simulink model "lab1_SimulinkExtendedStateEstimator"  (R2020b)
settings: Solver=VariableStepAuto  StartTime=0.0  StopTime=10.0  RelTol=1e-3
undefined symbols (not defined in the file): A_hat_e, A_r, A_r_2, A_r_3, B_e, C_p, enable_Reference, K, L_e, sens, w_1, w_2
settings Model: Creator=Musta  LastModifiedBy=Musta

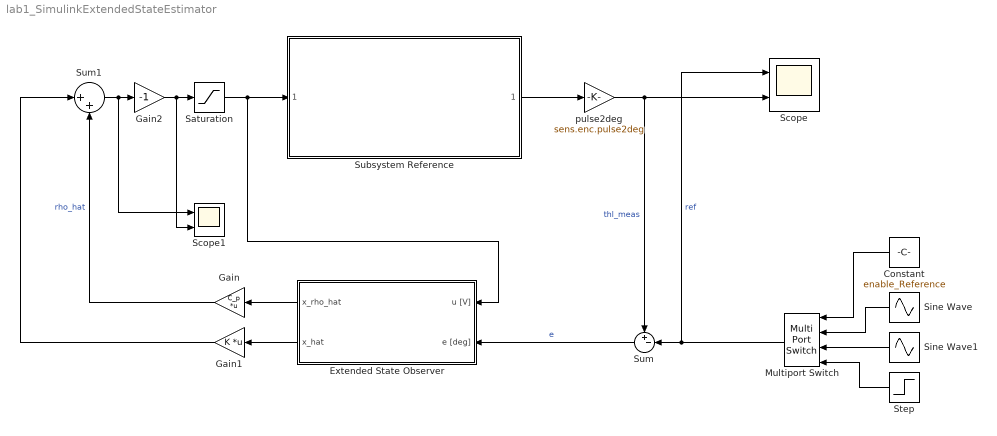
== system lab1_SimulinkExtendedStateEstimator ==
  Constant : Constant  Value=enable_Reference
  Extended State Observer : Subsystem
  Gain : Gain  Gain=C_p  Multiplication=Matrix(K*u)
  Gain1 : Gain  Gain=K  Multiplication=Matrix(K*u)
  Gain2 : Gain  Gain=-1
  Multiport Switch : MultiPortSwitch
  Saturation : Saturate  UpperLimit=10  LowerLimit=-10
  Scope : Scope  NumInputPorts=2
  Scope1 : Scope  NumInputPorts=2
  Sine Wave : Sin  Amplitude=A_r  Frequency=w_1  SampleTime=0
  Sine Wave1 : Sin  Amplitude=A_r_2  Frequency=w_2  SampleTime=0
  Step : Step  Time=0  After=A_r_3  SampleTime=0
  Subsystem Reference : Subsystem  ReferencedSubsystem=plant_Model
  Sum : Sum  Inputs=+-|
  Sum1 : Sum  Inputs=|++
  pulse2deg : Gain  Gain=sens.enc.pulse2deg
  wires:
  Multiport Switch/1 -> Scope/1, Sum/2  "ref"
  Sum1/1 -> Gain2/1, Scope1/1
  Sum/1 -> Extended State Observer/2(e [deg])  "e"
  pulse2deg/1 -> Sum/1, Scope/2  "thl_meas"
  Extended State Observer/1(x_rho_hat) -> Gain/1
  Gain/1 -> Sum1/2  "rho_hat"
  Extended State Observer/2(x_hat) -> Gain1/1
  Gain1/1 -> Sum1/1
  Saturation/1 -> Subsystem Reference/1, Extended State Observer/1(u [V])
  Gain2/1 -> Scope1/2, Saturation/1
  Subsystem Reference/1 -> pulse2deg/1
  Sine Wave/1 -> Multiport Switch/2
  Sine Wave1/1 -> Multiport Switch/3
  Step/1 -> Multiport Switch/4
  Constant/1 -> Multiport Switch/1

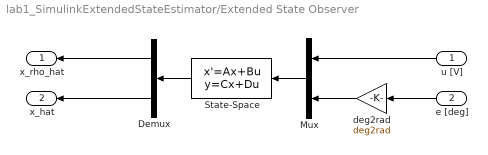
== system lab1_SimulinkExtendedStateEstimator/Extended State Observer ==
  u [V] : Inport
  e [deg] : Inport  Port=2
  Demux : Demux  Outputs=[3,2]
  Mux : Mux  Inputs=[1,1]
  State-Space : StateSpace  A=A_hat_e  B=[B_e L_e]  C=eye(5)  D=zeros(5,2)  InitialCondition=0
  deg2rad : Gain  Gain=deg2rad
  x_rho_hat : Outport
  x_hat : Outport  Port=2
  wires:
  e [deg]/1 -> deg2rad/1
  Demux/2 -> x_hat/1
  deg2rad/1 -> Mux/2
  State-Space/1 -> Demux/1
  Mux/1 -> State-Space/1
  Demux/1 -> x_rho_hat/1
  u [V]/1 -> Mux/1
